simulink model "pointing_group24"  (R2023b)
settings: Solver=FixedStepAuto  StartTime=0.0  StopTime=T  RelTol=1e-3
values from neighbouring files (symbols this model uses):
  a = 6939    [Air_Drag_script.m]    (also in main.m = 6939.063; main_group24.m = 6978)
  AccMagn = 0.5    [main_group24.m]
  AccSunSens = 0.125    [main_group24.m]
  ARW = deg2rad(0.10)    [main_group24.m]
  by = 0.1    [main_group24.m]
  bz = 0.1    [main_group24.m]
  c = 2.99792*10^8    (= 299792000)    [main.m]    (also in main_group24.m = 299792458)
  Cd = 2.2    [main_group24.m]
  e = 0    [Air_Drag_script.m]    (also in main.m = 0.001304; main_group24.m)
  G = [gn, gm, gvali, gsvi]    [main.m]    (also in main_group24.m)
  GyroSampleRate = 10    [main_group24.m]
  H = [hn, hm, hvali, hsvi]    [main.m]    (also in main_group24.m)
  H_0 = ((g1_0^2)+(g1_1^2)+(h1_1^2))^0.5    (= 2.98059244128e-05)    [main_group24.m]
  i = deg2rad(97.5307)    [Air_Drag_script.m]    (also in main.m; main_group24.m = deg2rad(98))
  I_tot = [Ix 0 0; 0 Iy 0; 0 0 Iz]    [data_mass.m]    (also in main_group24.m)
  invI_tot = inv(I_tot)    [data_mass.m]    (also in main_group24.m)
  Ix = J(1,1)    [Air_Drag_script.m]    (also in data_mass.m = 0.0755003333333; main.m = 0.057749855; main_group24.m = 0.0755003333333)
  Iy = J(2,2)    [Air_Drag_script.m]    (also in data_mass.m = 0.0755003333333; main.m = 0.04143542; main_group24.m = 0.0755003333333)
  Iz = J(3,3)    [Air_Drag_script.m]    (also in data_mass.m = 0.055; main.m = 0.024624309; main_group24.m = 0.055)
  k1 = 5e-2    (= 0.05)    [main_group24.m]
  k2 = 2.5e-2    (= 0.025)    [main_group24.m]
  m = [0.1; 0.1; 0.1]    [main.m]    (also in main_group24.m)
  MB = [4; 0.1; 0.1; 0.3]    [main.m]    (also in main_group24.m)
  MMnoise = 15e-9*[1; 1; 1]    [main_group24.m]
  MMSampleRate = 1    [main_group24.m]
  mu = 3.98600433e+5    (= 398600.433)    [main.m]    (also in main_group24.m)
  n = 0.0011    [Air_Drag_script.m]    (also in main.m = sqrt(mu/a^3); main_group24.m = sqrt(mu/a^3))
  n_E = 729.2e-07    (= 7.292e-05)    [main_group24.m]
  om_E = 0.000072921    (= 7.2921e-05)    [main_group24.m]
  P = Fe/c    (= 4.52980041279e-06)    [main_group24.m]
  q0 = [ 1 1 1 1 ]'    [Air_Drag_script.m]    (also in main_group24.m = [0 0 0 1]')
  R_e = 6378    [main.m]    (also in main_group24.m)
  rho_air = 1.65e-13    [Air_Drag_script.m]    (also in main_group24.m = 6.967e-13)
  rho_d_body = 0.1*2/3    (= 0.0666666666667)    [main_group24.m]
  rho_d_sp = 0.1*2/3    (= 0.0666666666667)    [main_group24.m]
  rho_s_body = 0.5    [main_group24.m]
  rho_s_sp = 0.1    [main_group24.m]
  RRW = deg2rad(0.3)    [main_group24.m]
  SP = [1; 0.3; 0.1; 0.01]    [main.m]    (also in main_group24.m = [0.25; 0.1; 0.3; 0.01])
undefined symbols (not defined in the file or in its folder): pan, s1, s2, s3, s4, s5, s6, thrust
libraries: vrlib x25, matrix_library x17, simulink_extras x8, sharedutil x3, simulink x1
(part 3 of 5)

== system pointing_group24/Desturbances/External Torques/Reflected radiation/Force MB/Subsystem ==
  S_B : Inport
  N_MB : Inport  Port=2
  Constant3 : Constant  Value=[1, 1, 1]
  Matrix Multiply5 : Product  Multiplication=Matrix(*)
  Product10 : Product
  Reshape11 : Reshape  OutputDimensionality=Row vector (2-D)
  Reshape12 : Reshape  OutputDimensionality=Column vector (2-D)
  Sum of Elements : Sum  Inputs=+  CollapseMode=Specified dimension  CollapseDim=2
  Out1 : Outport
  wires:
  Reshape11/1 -> Matrix Multiply5/2
  Constant3/1 -> Reshape11/1
  Sum of Elements/1 -> Out1/1
  N_MB/1 -> Product10/2
  Product10/1 -> Sum of Elements/1
  S_B/1 -> Reshape12/1
  Reshape12/1 -> Matrix Multiply5/1
  Matrix Multiply5/1 -> Product10/1

== system pointing_group24/Desturbances/External Torques/Reflected radiation/SP center arm/r_SPx ==
  b_SP : Inport
  a_MB : Inport  Port=2
  Constant : Constant  Value=[1 0 0]
  Gain : Gain  Gain=1/2
  Gain1 : Gain  Gain=1/2
  Gain2 : Gain  Gain=-1
  Product : Product
  Reshape : Reshape  OutputDimensionality=Column vector (2-D)
  Sum : Sum
  r_SP1 : Outport
  r_SP2 : Outport  Port=2
  wires:
  Product/1 -> Gain2/1, r_SP1/1
  Gain2/1 -> r_SP2/1
  Sum/1 -> Product/2
  Reshape/1 -> Product/1
  Gain/1 -> Sum/2
  Gain1/1 -> Sum/1
  b_SP/1 -> Gain1/1
  a_MB/1 -> Gain/1
  Constant/1 -> Reshape/1

== system pointing_group24/Desturbances/External Torques/Reflected radiation/SP center arm/r_SPy ==
  b_SP : Inport
  b_MB : Inport  Port=2
  Constant : Constant  Value=[0 1 0]
  Gain : Gain  Gain=1/2
  Gain1 : Gain  Gain=1/2
  Gain2 : Gain  Gain=-1
  Product : Product
  Reshape : Reshape  OutputDimensionality=Column vector (2-D)
  Sum : Sum
  r_SP1 : Outport
  r_SP2 : Outport  Port=2
  wires:
  Constant/1 -> Reshape/1
  b_MB/1 -> Gain/1
  b_SP/1 -> Gain1/1
  Gain1/1 -> Sum/1
  Gain/1 -> Sum/2
  Reshape/1 -> Product/1
  Sum/1 -> Product/2
  Gain2/1 -> r_SP2/1
  Product/1 -> r_SP1/1, Gain2/1

== system pointing_group24/Desturbances/External Torques/Reflected radiation/S_B dot N_MB/If Action Subsystem ==
  NMB : Inport
  Action Port : ActionPort  ActionPortLabel=if(u1 > 0)
  Constant : Constant
  Selector : Selector  NumberOfDimensions=2  InputPortWidth=3  IndexOptions=Index vector (dialog),Index vector (dialog)  Indices=1,[1 2 3]  OutputSizes=1,1
  x : Outport
  pointer : Outport  Port=2
  wires:
  Constant/1 -> pointer/1
  Selector/1 -> x/1
  NMB/1 -> Selector/1

== system pointing_group24/Desturbances/External Torques/Reflected radiation/S_B dot N_MB/If Action Subsystem1 ==
  NMB : Inport
  Action Port : ActionPort  ActionPortLabel=if(u1 > 0)
  Constant : Constant
  Selector : Selector  NumberOfDimensions=2  InputPortWidth=3  IndexOptions=Index vector (dialog),Index vector (dialog)  Indices=2,[1 2 3]  OutputSizes=1,1
  y : Outport
  pointer : Outport  Port=2
  wires:
  Constant/1 -> pointer/1
  NMB/1 -> Selector/1
  Selector/1 -> y/1

== system pointing_group24/Desturbances/External Torques/Reflected radiation/S_B dot N_MB/If Action Subsystem2 ==
  NMB : Inport
  Action Port : ActionPort  ActionPortLabel=if(u1 > 0)
  Constant : Constant
  Selector : Selector  NumberOfDimensions=2  InputPortWidth=3  IndexOptions=Index vector (dialog),Index vector (dialog)  Indices=3,[1 2 3]  OutputSizes=1,1
  z : Outport
  pointer : Outport  Port=2
  wires:
  Constant/1 -> pointer/1
  Selector/1 -> z/1
  NMB/1 -> Selector/1

== system pointing_group24/Desturbances/External Torques/Reflected radiation/S_B dot N_MB/If Action Subsystem3 ==
  NMB : Inport
  Action Port : ActionPort  ActionPortLabel=else
  Constant : Constant  Value=-1
  Selector : Selector  NumberOfDimensions=2  InputPortWidth=3  IndexOptions=Index vector (dialog),Index vector (dialog)  Indices=4,[1 2 3]  OutputSizes=1,1
  -x : Outport
  pointer : Outport  Port=2
  wires:
  Constant/1 -> pointer/1
  NMB/1 -> Selector/1
  Selector/1 -> -x/1

== system pointing_group24/Desturbances/External Torques/Reflected radiation/S_B dot N_MB/If Action Subsystem4 ==
  NMB : Inport
  Action Port : ActionPort  ActionPortLabel=else
  Constant : Constant  Value=-1
  Selector : Selector  NumberOfDimensions=2  InputPortWidth=3  IndexOptions=Index vector (dialog),Index vector (dialog)  Indices=5,[1 2 3]  OutputSizes=1,1
  -y : Outport
  pointer : Outport  Port=2
  wires:
  Constant/1 -> pointer/1
  Selector/1 -> -y/1
  NMB/1 -> Selector/1

== system pointing_group24/Desturbances/External Torques/Reflected radiation/S_B dot N_MB/If Action Subsystem5 ==
  NMB : Inport
  Action Port : ActionPort  ActionPortLabel=else
  Constant : Constant  Value=-1
  Selector : Selector  NumberOfDimensions=2  InputPortWidth=3  IndexOptions=Index vector (dialog),Index vector (dialog)  Indices=6,[1 2 3]  OutputSizes=1,1
  -z : Outport
  pointer : Outport  Port=2
  wires:
  Constant/1 -> pointer/1
  NMB/1 -> Selector/1
  Selector/1 -> -z/1

== system pointing_group24/Desturbances/External Torques/Reflected radiation/S_B dot N_SP/If Action Subsystem ==
  N_SP : Inport
  Action Port : ActionPort  ActionPortLabel=if(u1 > 0)
  Constant : Constant
  Selector : Selector  NumberOfDimensions=2  InputPortWidth=3  IndexOptions=Index vector (dialog),Index vector (dialog)  Indices=1,[1 2 3]  OutputSizes=1,1
  true_NSP : Outport
  pointer : Outport  Port=2
  wires:
  Selector/1 -> true_NSP/1
  Constant/1 -> pointer/1
  N_SP/1 -> Selector/1

== system pointing_group24/Desturbances/External Torques/Reflected radiation/S_B dot N_SP/If Action Subsystem1 ==
  N_SP : Inport
  Action Port : ActionPort  ActionPortLabel=if(u1 > 0)
  Constant : Constant  Value=-1
  Selector : Selector  NumberOfDimensions=2  InputPortWidth=3  IndexOptions=Index vector (dialog),Index vector (dialog)  Indices=2,[1 2 3]  OutputSizes=1,1
  true_NSP : Outport
  pointer : Outport  Port=2
  wires:
  N_SP/1 -> Selector/1
  Constant/1 -> pointer/1
  Selector/1 -> true_NSP/1

== system pointing_group24/Desturbances/External Torques/Reflected radiation/Torque arm MB/creazione raggi vettore tra CM MB e centro facce illuminate della faccia che ha come normale l'asse i ==
  S_B : Inport
  MB : Inport  Port=2
  A_vect : Inport  Port=3
  pointer : Inport  Port=4
  Add2 : Sum  Inputs=+|+|+|+|+
  Demux1 : Demux  Outputs=3
  If Action Subsystem : Subsystem  TreatAsAtomicUnit=on
  If Action Subsystem1 : Subsystem  TreatAsAtomicUnit=on
  If Action Subsystem2 : Subsystem  TreatAsAtomicUnit=on
  If Action Subsystem3 : Subsystem  TreatAsAtomicUnit=on
  If Action Subsystem4 : Subsystem  TreatAsAtomicUnit=on
  If Action Subsystem5 : Subsystem  TreatAsAtomicUnit=on
  If Action Subsystem6 : Subsystem  TreatAsAtomicUnit=on
  If Action Subsystem8 : Subsystem  TreatAsAtomicUnit=on
  If1 : If  NumInputs=2  IfExpression=u1>0 & u2>0
  If2 : If  NumInputs=2  IfExpression=u1<0 & u2>0
  If3 : If  NumInputs=2  IfExpression=u1>0 & u2<0
  If4 : If  NumInputs=2  IfExpression=u1<0 & u2<0
  Merge{,1..3} (4 alike) : Merge
  Reshape1 : Reshape  OutputDimensionality=Column vector (2-D)
  Terminator1 : Terminator
  creating distance between cm MB and centro geom lato : Subsystem
  Out1 : Outport
  wires:
  pointer/1 -> creating distance between cm MB and centro geom lato/2(pointer)
  A_vect/1 -> [A_vect]
  [MB] -> creating distance between cm MB and centro geom lato/1(MB)
  If Action Subsystem6/1(Out1) -> Merge3/2
  Merge2/1 -> Add2/4  "raggio vettore centro geom lato- centro geom lato illuminato"
  If Action Subsystem5/1(Out1) -> Merge2/2
  If Action Subsystem1/1(r_cface_cluce_yneg_z_pos) -> Merge2/1
  If Action Subsystem3/1(Out1) -> Merge1/2
  If4/2 -> If Action Subsystem6/Action
  If3/2 -> If Action Subsystem5/Action
  If2/2 -> If Action Subsystem3/Action
  If Action Subsystem8/1(Out1) -> Merge/2
  [MB] -> If Action Subsystem2/2(MB)
  [MB] -> If Action Subsystem1/2(MB)
  [MB] -> If Action Subsystem4/2(MB)
  [MB] -> If Action Subsystem/2(MB)
  MB/1 -> [MB]
  Demux1/1 -> Terminator1/1  "S_B_x"
  creating distance between cm MB and centro geom lato/1(Out1) -> Add2/1
  Demux1/3 -> If1/1, If2/1, If3/1, If4/1  "S_B_z"
  If1/1 -> If Action Subsystem/Action
  If2/1 -> If Action Subsystem4/Action
  Demux1/2 -> If1/2, If4/2, If3/2, If2/2  "S_B_y"
  Reshape1/1 -> Demux1/1
  S_B/1 -> Reshape1/1
  If1/2 -> If Action Subsystem8/Action
  If Action Subsystem/1(r_cface_cluce_yz_pos) -> Merge/1
  Merge/1 -> Add2/2  "raggio vettore centro geom lato- centro geom lato illuminato"
  If Action Subsystem4/1(r_cface_cluce_zneg_y_pos) -> Merge1/1
  Merge1/1 -> Add2/3  "raggio vettore centro geom lato- centro geom lato illuminato"
  [A_vect] -> If Action Subsystem/1(Areas_vect)
  If3/1 -> If Action Subsystem1/Action
  If Action Subsystem2/1(r_cface_cluce_yneg_z_neg) -> Merge3/1
  If4/1 -> If Action Subsystem2/Action
  Merge3/1 -> Add2/5  "raggio vettore centro geom lato- centro geom lato illuminato"
  Add2/1 -> Out1/1
  [A_vect] -> If Action Subsystem4/1(Areas_vect)
  [A_vect] -> If Action Subsystem1/1(Areas_vect)
  [A_vect] -> If Action Subsystem2/1(Areas_vect)

== system pointing_group24/Desturbances/External Torques/Reflected radiation/Torque arm MB/creazione raggi vettore tra CM MB e centro facce illuminate della faccia che ha come normale l'asse j ==
  S_B : Inport
  MB : Inport  Port=2
  A_vect : Inport  Port=3
  pointer : Inport  Port=4
  Add2 : Sum  Inputs=+|+|+|+|+
  Demux1 : Demux  Outputs=3
  If Action Subsystem : Subsystem  TreatAsAtomicUnit=on
  If Action Subsystem1 : Subsystem  TreatAsAtomicUnit=on
  If Action Subsystem2 : Subsystem  TreatAsAtomicUnit=on
  If Action Subsystem3 : Subsystem  TreatAsAtomicUnit=on
  If Action Subsystem4 : Subsystem  TreatAsAtomicUnit=on
  If Action Subsystem5 : Subsystem  TreatAsAtomicUnit=on
  If Action Subsystem6 : Subsystem  TreatAsAtomicUnit=on
  If Action Subsystem7 : Subsystem  TreatAsAtomicUnit=on
  If1 : If  NumInputs=2  IfExpression=u1>0 & u2>0
  If2 : If  NumInputs=2  IfExpression=u1<0 & u2>0
  If3 : If  NumInputs=2  IfExpression=u1>0 & u2<0
  If4 : If  NumInputs=2  IfExpression=u1<0 & u2<0
  Merge{,1..3} (4 alike) : Merge
  Reshape1 : Reshape  OutputDimensionality=Column vector (2-D)
  Terminator1 : Terminator
  creating distance between cm MB and centro geom lato1 : Subsystem
  Out1 : Outport
  wires:
  pointer/1 -> creating distance between cm MB and centro geom lato1/2(pointer)
  A_vect/1 -> [A_vect]
  [MB] -> creating distance between cm MB and centro geom lato1/1(MB)
  If Action Subsystem7/1(Out1) -> Merge3/2
  If Action Subsystem6/1(Out1) -> Merge2/2
  If Action Subsystem2/1(r_cface_cluce_x_neg_z_pos) -> Merge2/1
  If Action Subsystem4/1(Out1) -> Merge1/2
  If Action Subsystem5/1(Out1) -> Merge/2
  If4/2 -> If Action Subsystem7/Action
  If3/2 -> If Action Subsystem6/Action
  If2/2 -> If Action Subsystem4/Action
  If1/2 -> If Action Subsystem5/Action
  [MB] -> If Action Subsystem3/2(MB)
  [MB] -> If Action Subsystem2/2(MB)
  [MB] -> If Action Subsystem1/2(MB)
  [MB] -> If Action Subsystem/2(MB)
  MB/1 -> [MB]
  Demux1/1 -> If2/2, If3/2, If4/2, If1/2  "S_B_x"
  Demux1/3 -> If1/1, If2/1, If3/1, If4/1  "S_B_z"
  [A_vect] -> If Action Subsystem3/1(Areas_vect)
  [A_vect] -> If Action Subsystem2/1(Areas_vect)
  [A_vect] -> If Action Subsystem1/1(Areas_vect)
  Add2/1 -> Out1/1
  Merge3/1 -> Add2/5  "raggio vettore centro geom lato- centro geom lato illuminato"
  If4/1 -> If Action Subsystem3/Action
  If Action Subsystem3/1(r_cface_cluce_x_neg_z_neg) -> Merge3/1
  If3/1 -> If Action Subsystem2/Action
  Merge2/1 -> Add2/4  "raggio vettore centro geom lato- centro geom lato illuminato"
  [A_vect] -> If Action Subsystem/1(Areas_vect)
  Merge1/1 -> Add2/3  "raggio vettore centro geom lato- centro geom lato illuminato"
  If Action Subsystem1/1(r_cface_cluce_x_pos_z_neg) -> Merge1/1
  Merge/1 -> Add2/2  "raggio vettore centro geom lato- centro geom lato illuminato"
  If Action Subsystem/1(r_cface_cluce_xz_pos) -> Merge/1
  S_B/1 -> Reshape1/1
  Reshape1/1 -> Demux1/1
  If2/1 -> If Action Subsystem1/Action
  If1/1 -> If Action Subsystem/Action
  creating distance between cm MB and centro geom lato1/1(Out1) -> Add2/1
  Demux1/2 -> Terminator1/1

== system pointing_group24/Desturbances/External Torques/Reflected radiation/Torque arm MB/creazione raggi vettore tra CM MB e centro facce illuminate della faccia che ha come normale l'asse k ==
  S_B : Inport
  MB : Inport  Port=2
  A_vect : Inport  Port=3
  pointer : Inport  Port=4
  Add2 : Sum  Inputs=+|+|+|+|+
  Demux1 : Demux  Outputs=3
  If Action Subsystem : Subsystem  TreatAsAtomicUnit=on
  If Action Subsystem1 : Subsystem  TreatAsAtomicUnit=on
  If Action Subsystem2 : Subsystem  TreatAsAtomicUnit=on
  If Action Subsystem3 : Subsystem  TreatAsAtomicUnit=on
  If Action Subsystem4 : Subsystem  TreatAsAtomicUnit=on
  If Action Subsystem5 : Subsystem  TreatAsAtomicUnit=on
  If Action Subsystem6 : Subsystem  TreatAsAtomicUnit=on
  If Action Subsystem7 : Subsystem  TreatAsAtomicUnit=on
  If1 : If  NumInputs=2  IfExpression=u1>0 & u2>0
  If2 : If  NumInputs=2  IfExpression=u1<0 & u2>0
  If3 : If  NumInputs=2  IfExpression=u1>0 & u2<0
  If4 : If  NumInputs=2  IfExpression=u1<0 & u2<0
  Merge{,1..3} (4 alike) : Merge
  Reshape1 : Reshape  OutputDimensionality=Column vector (2-D)
  Terminator1 : Terminator
  creating distance between cm MB and centro geom lato1 : Subsystem
  Out1 : Outport
  wires:
  pointer/1 -> creating distance between cm MB and centro geom lato1/2(pointer)
  A_vect/1 -> [A_vect]
  creating distance between cm MB and centro geom lato1/1(Out1) -> Add2/1
  [MB] -> creating distance between cm MB and centro geom lato1/1(MB)
  If Action Subsystem7/1(Out1) -> Merge3/2
  If Action Subsystem2/1(r_cface_cluce_xneg_y_neg) -> Merge3/1
  If Action Subsystem6/1(Out1) -> Merge2/2
  If Action Subsystem3/1(Out1) -> Merge1/2
  If Action Subsystem4/1(r_cface_cluce_xneg_y_pos) -> Merge1/1
  If Action Subsystem5/1(Out1) -> Merge/2
  If Action Subsystem/1(r_cface_cluce_xy_pos) -> Merge/1
  If2/2 -> If Action Subsystem3/Action
  [MB] -> If Action Subsystem2/2(MB1)
  [MB] -> If Action Subsystem1/2(MB)
  [MB] -> If Action Subsystem4/2(MB1)
  [MB] -> If Action Subsystem/2(MB)
  MB/1 -> [MB]
  [A_vect] -> If Action Subsystem2/1(Areas_vect)
  [A_vect] -> If Action Subsystem1/1(Areas_vect)
  [A_vect] -> If Action Subsystem4/1(Areas_vect)
  Add2/1 -> Out1/1
  Merge3/1 -> Add2/5  "raggio vettore centro geom lato- centro geom lato illuminato"
  If4/1 -> If Action Subsystem2/Action
  If4/2 -> If Action Subsystem7/Action
  If3/1 -> If Action Subsystem1/Action
  If Action Subsystem1/1(r_cface_cluce_xpos_y_neg) -> Merge2/1
  If3/2 -> If Action Subsystem6/Action
  Merge2/1 -> Add2/4  "raggio vettore centro geom lato- centro geom lato illuminato"
  [A_vect] -> If Action Subsystem/1(Areas_vect)
  Merge1/1 -> Add2/3  "raggio vettore centro geom lato- centro geom lato illuminato"
  Merge/1 -> Add2/2  "raggio vettore centro geom lato- centro geom lato illuminato"
  If1/2 -> If Action Subsystem5/Action
  S_B/1 -> Reshape1/1
  Reshape1/1 -> Demux1/1
  Demux1/2 -> If1/2, If2/2, If3/2, If4/2  "S_B_y"
  If2/1 -> If Action Subsystem4/Action
  If1/1 -> If Action Subsystem/Action
  Demux1/1 -> If2/1, If3/1, If4/1, If1/1  "S_B_x"
  Demux1/3 -> Terminator1/1

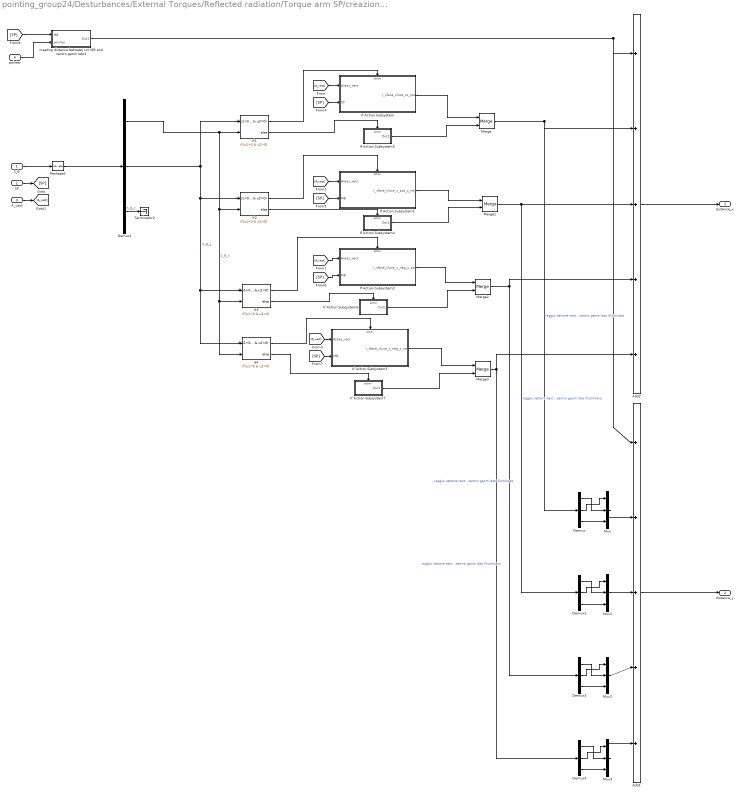
== system pointing_group24/Desturbances/External Torques/Reflected radiation/Torque arm SP/creazione raggi vettore tra CM SP e centro di pressione della faccia illuminata ==
  S_B : Inport
  SP : Inport  Port=2
  A_vect : Inport  Port=3
  pointer : Inport  Port=4
  Add1 : Sum  Inputs=+|+|+|+|+
  Add2 : Sum  Inputs=+|+|+|+|+
  Demux{,1..4} (5 alike) : Demux  Outputs=3
  If Action Subsystem : Subsystem  TreatAsAtomicUnit=on
  If Action Subsystem1 : Subsystem  TreatAsAtomicUnit=on
  If Action Subsystem2 : Subsystem  TreatAsAtomicUnit=on
  If Action Subsystem3 : Subsystem  TreatAsAtomicUnit=on
  If Action Subsystem4 : Subsystem  TreatAsAtomicUnit=on
  If Action Subsystem5 : Subsystem  TreatAsAtomicUnit=on
  If Action Subsystem6 : Subsystem  TreatAsAtomicUnit=on
  If Action Subsystem7 : Subsystem  TreatAsAtomicUnit=on
  If1 : If  NumInputs=2  IfExpression=u1>0 & u2>0
  If2 : If  NumInputs=2  IfExpression=u1<0 & u2>0
  If3 : If  NumInputs=2  IfExpression=u1>0 & u2<0
  If4 : If  NumInputs=2  IfExpression=u1<0 & u2<0
  Merge{,1..3} (4 alike) : Merge
  Mux{,1..3} (4 alike) : Mux  Inputs=3
  Reshape1 : Reshape  OutputDimensionality=Column vector (2-D)
  Terminator2 : Terminator
  creating distance between cm MB and centro geom lato1 : Subsystem
  distance_x : Outport
  distance_y : Outport  Port=2
  wires:
  Mux2/1 -> Add1/4
  Mux3/1 -> Add1/5
  Demux4/1 -> Mux3/2
  Demux4/2 -> Mux3/1
  Demux4/3 -> Mux3/3
  Demux3/3 -> Mux2/3
  Demux3/2 -> Mux2/1
  Demux3/1 -> Mux2/2
  Demux2/1 -> Mux1/2
  Demux2/2 -> Mux1/1
  Demux2/3 -> Mux1/3
  Mux1/1 -> Add1/3
  Mux/1 -> Add1/2
  Demux/3 -> Mux/3
  Demux/2 -> Mux/1
  Demux/1 -> Mux/2
  Add1/1 -> distance_y/1
  Demux1/3 -> Terminator2/1  "S_B_z"
  pointer/1 -> creating distance between cm MB and centro geom lato1/2(pointer)
  A_vect/1 -> [A_vect]
  [SP] -> creating distance between cm MB and centro geom lato1/1(MB)
  If Action Subsystem7/1(Out1) -> Merge3/2
  If Action Subsystem6/1(Out1) -> Merge2/2
  If Action Subsystem2/1(r_cface_cluce_x_neg_z_pos) -> Merge2/1
  If Action Subsystem4/1(Out1) -> Merge1/2
  If Action Subsystem5/1(Out1) -> Merge/2
  If4/2 -> If Action Subsystem7/Action
  If3/2 -> If Action Subsystem6/Action
  If2/2 -> If Action Subsystem4/Action
  If1/2 -> If Action Subsystem5/Action
  [SP] -> If Action Subsystem3/2(MB)
  [SP] -> If Action Subsystem2/2(MB)
  [SP] -> If Action Subsystem1/2(MB)
  [SP] -> If Action Subsystem/2(SP)
  SP/1 -> [SP]
  Demux1/1 -> If2/2, If3/2, If4/2, If1/2  "S_B_x"
  Demux1/2 -> If1/1, If2/1, If3/1, If4/1  "S_B_y"
  [A_vect] -> If Action Subsystem3/1(Areas_vect)
  [A_vect] -> If Action Subsystem2/1(Areas_vect)
  [A_vect] -> If Action Subsystem1/1(Areas_vect)
  Add2/1 -> distance_x/1
  Merge3/1 -> Add2/5, Demux4/1  "raggio vettore centro geom lato- centro geom lato illuminato"
  If4/1 -> If Action Subsystem3/Action
  If Action Subsystem3/1(r_cface_cluce_x_neg_z_neg) -> Merge3/1
  If3/1 -> If Action Subsystem2/Action
  Merge2/1 -> Add2/4, Demux3/1  "raggio vettore centro geom lato- centro geom lato illuminato"
  [A_vect] -> If Action Subsystem/1(Areas_vect)
  Merge1/1 -> Add2/3, Demux2/1  "raggio vettore centro geom lato- centro geom lato illuminato"
  If Action Subsystem1/1(r_cface_cluce_x_pos_z_neg) -> Merge1/1
  Merge/1 -> Add2/2, Demux/1  "raggio vettore centro geom lato- centro geom lato illuminato"
  If Action Subsystem/1(r_cface_cluce_xz_pos) -> Merge/1
  S_B/1 -> Reshape1/1
  Reshape1/1 -> Demux1/1
  If2/1 -> If Action Subsystem1/Action
  If1/1 -> If Action Subsystem/Action
  creating distance between cm MB and centro geom lato1/1(Out1) -> Add2/1, Add1/1

== system pointing_group24/Desturbances/External Torques/SRP con frecce/SRP/Subsystem ==
  S_B : Inport
  Add22 : Sum
  Add23 : Sum
  Add24 : Sum  Inputs=+-
  Constant30 : Constant  Value=s2.A
  Constant31 : Constant  Value=s2.n
  Constant44 : Constant  Value=rho_d_body
  Constant47 : Constant  Value=s2.n
  Constant50 : Constant
  Constant51 : Constant  Value=rho_s_body
  Constant52 : Constant  Value=s2.r
  Cross Product10 : vrlib/Utilities/Cross Product
  Dot Product10 : DotProduct  OutDataTypeStr=Inherit: Inherit via internal rule
  Gain40 : Gain  Gain=0
  Gain41 : Gain  Gain=-P
  Gain42 : Gain  Gain=2
  Gain43 : Gain  Gain=rho_s_body
  Product{1..4} (4 alike) : Product
  Switch10 : Switch  Criteria=u2 > Threshold  SaturateOnIntegerOverflow=off  InputSameDT=off
  pan2 : Outport
  wires:
  Constant50/1 -> Add24/1
  Gain42/1 -> Gain43/1
  Cross Product10/1 -> pan2/1
  Gain43/1 -> Add22/2
  Constant52/1 -> Cross Product10/1
  Add22/1 -> Product2/2
  Gain41/1 -> Product1/2
  Gain40/1 -> Switch10/3
  Dot Product10/1 -> Gain40/1, Switch10/1, Switch10/2
  Product2/1 -> Add23/2
  Constant31/1 -> Dot Product10/2
  Constant51/1 -> Add24/2
  Add24/1 -> Product3/2
  Product3/1 -> Add23/1
  Constant44/1 -> Add22/1
  S_B/1 -> Product3/1, Dot Product10/1
  Product1/1 -> Product4/1
  Constant47/1 -> Product2/1
  Switch10/1 -> Gain41/1, Gain42/1
  Constant30/1 -> Product1/1
  Product4/1 -> Cross Product10/2
  Add23/1 -> Product4/2

== system pointing_group24/Desturbances/External Torques/SRP con frecce/SRP/Subsystem1 ==
  S_B : Inport
  Add22 : Sum
  Add23 : Sum
  Add24 : Sum  Inputs=+-
  Constant30 : Constant  Value=s3.A
  Constant31 : Constant  Value=s3.n
  Constant44 : Constant  Value=rho_d_body
  Constant47 : Constant  Value=s3.n
  Constant50 : Constant
  Constant51 : Constant  Value=rho_s_body
  Constant52 : Constant  Value=s3.r
  Cross Product10 : vrlib/Utilities/Cross Product
  Dot Product10 : DotProduct  OutDataTypeStr=Inherit: Inherit via internal rule
  Gain40 : Gain  Gain=0
  Gain41 : Gain  Gain=-P
  Gain42 : Gain  Gain=2
  Gain43 : Gain  Gain=rho_s_body
  Product{1..4} (4 alike) : Product
  Switch10 : Switch  Criteria=u2 > Threshold  SaturateOnIntegerOverflow=off  InputSameDT=off
  pan3 : Outport
  wires:
  Add23/1 -> Product4/2
  Product4/1 -> Cross Product10/2
  Constant30/1 -> Product1/1
  Switch10/1 -> Gain42/1, Gain41/1
  Constant47/1 -> Product2/1
  Product1/1 -> Product4/1
  S_B/1 -> Dot Product10/1, Product3/1
  Constant44/1 -> Add22/1
  Product3/1 -> Add23/1
  Add24/1 -> Product3/2
  Constant51/1 -> Add24/2
  Constant31/1 -> Dot Product10/2
  Product2/1 -> Add23/2
  Dot Product10/1 -> Switch10/2, Switch10/1, Gain40/1
  Gain40/1 -> Switch10/3
  Gain41/1 -> Product1/2
  Add22/1 -> Product2/2
  Constant52/1 -> Cross Product10/1
  Gain43/1 -> Add22/2
  Cross Product10/1 -> pan3/1
  Gain42/1 -> Gain43/1
  Constant50/1 -> Add24/1

== system pointing_group24/Desturbances/External Torques/SRP con frecce/SRP/Subsystem2 ==
  S_B : Inport
  Add22 : Sum
  Add23 : Sum
  Add24 : Sum  Inputs=+-
  Constant30 : Constant  Value=s1.A
  Constant31 : Constant  Value=s1.n
  Constant44 : Constant  Value=rho_d_body
  Constant47 : Constant  Value=s1.n
  Constant50 : Constant
  Constant51 : Constant  Value=rho_s_body
  Constant52 : Constant  Value=s1.r
  Cross Product10 : vrlib/Utilities/Cross Product
  Dot Product10 : DotProduct  OutDataTypeStr=Inherit: Inherit via internal rule
  Gain40 : Gain  Gain=0
  Gain41 : Gain  Gain=-P
  Gain42 : Gain  Gain=2
  Gain43 : Gain  Gain=rho_s_body
  Product{1..4} (4 alike) : Product
  Switch10 : Switch  Criteria=u2 > Threshold  SaturateOnIntegerOverflow=off  InputSameDT=off
  pan1 : Outport
  wires:
  Add23/1 -> Product4/2
  Product4/1 -> Cross Product10/2
  Constant30/1 -> Product1/1
  Switch10/1 -> Gain42/1, Gain41/1
  Constant47/1 -> Product2/1
  Product1/1 -> Product4/1
  S_B/1 -> Dot Product10/1, Product3/1
  Constant44/1 -> Add22/1
  Product3/1 -> Add23/1
  Add24/1 -> Product3/2
  Constant51/1 -> Add24/2
  Constant31/1 -> Dot Product10/2
  Product2/1 -> Add23/2
  Dot Product10/1 -> Switch10/2, Switch10/1, Gain40/1
  Gain40/1 -> Switch10/3
  Gain41/1 -> Product1/2
  Add22/1 -> Product2/2
  Constant52/1 -> Cross Product10/1
  Gain43/1 -> Add22/2
  Cross Product10/1 -> pan1/1
  Gain42/1 -> Gain43/1
  Constant50/1 -> Add24/1

== system pointing_group24/Desturbances/External Torques/SRP con frecce/SRP/Subsystem3 ==
  S_B : Inport
  Add22 : Sum
  Add23 : Sum
  Add24 : Sum  Inputs=+-
  Constant30 : Constant  Value=s5.A
  Constant31 : Constant  Value=s5.n
  Constant44 : Constant  Value=rho_d_body
  Constant47 : Constant  Value=s5.n
  Constant50 : Constant
  Constant51 : Constant  Value=rho_s_body
  Constant52 : Constant  Value=s5.r
  Cross Product10 : vrlib/Utilities/Cross Product
  Dot Product10 : DotProduct  OutDataTypeStr=Inherit: Inherit via internal rule
  Gain40 : Gain  Gain=0
  Gain41 : Gain  Gain=-P
  Gain42 : Gain  Gain=2
  Gain43 : Gain  Gain=rho_s_body
  Product{1..4} (4 alike) : Product
  Switch10 : Switch  Criteria=u2 > Threshold  SaturateOnIntegerOverflow=off  InputSameDT=off
  pan5 : Outport
  wires:
  Constant50/1 -> Add24/1
  Gain42/1 -> Gain43/1
  Cross Product10/1 -> pan5/1
  Gain43/1 -> Add22/2
  Constant52/1 -> Cross Product10/1
  Add22/1 -> Product2/2
  Gain41/1 -> Product1/2
  Gain40/1 -> Switch10/3
  Dot Product10/1 -> Gain40/1, Switch10/1, Switch10/2
  Product2/1 -> Add23/2
  Constant31/1 -> Dot Product10/2
  Constant51/1 -> Add24/2
  Add24/1 -> Product3/2
  Product3/1 -> Add23/1
  Constant44/1 -> Add22/1
  S_B/1 -> Product3/1, Dot Product10/1
  Product1/1 -> Product4/1
  Constant47/1 -> Product2/1
  Switch10/1 -> Gain41/1, Gain42/1
  Constant30/1 -> Product1/1
  Product4/1 -> Cross Product10/2
  Add23/1 -> Product4/2

== system pointing_group24/Desturbances/External Torques/SRP con frecce/SRP/Subsystem4 ==
  S_B : Inport
  Add22 : Sum
  Add23 : Sum
  Add24 : Sum  Inputs=+-
  Constant30 : Constant  Value=s4.A
  Constant31 : Constant  Value=s4.n
  Constant44 : Constant  Value=rho_d_body
  Constant47 : Constant  Value=s4.n
  Constant50 : Constant
  Constant51 : Constant  Value=rho_s_body
  Constant52 : Constant  Value=s4.r
  Cross Product10 : vrlib/Utilities/Cross Product
  Dot Product10 : DotProduct  OutDataTypeStr=Inherit: Inherit via internal rule
  Gain40 : Gain  Gain=0
  Gain41 : Gain  Gain=-P
  Gain42 : Gain  Gain=2
  Gain43 : Gain  Gain=rho_s_body
  Product{1..4} (4 alike) : Product
  Switch10 : Switch  Criteria=u2 > Threshold  SaturateOnIntegerOverflow=off  InputSameDT=off
  pan4 : Outport
  wires:
  Constant50/1 -> Add24/1
  Gain42/1 -> Gain43/1
  Cross Product10/1 -> pan4/1
  Gain43/1 -> Add22/2
  Constant52/1 -> Cross Product10/1
  Add22/1 -> Product2/2
  Gain41/1 -> Product1/2
  Gain40/1 -> Switch10/3
  Dot Product10/1 -> Gain40/1, Switch10/1, Switch10/2
  Product2/1 -> Add23/2
  Constant31/1 -> Dot Product10/2
  Constant51/1 -> Add24/2
  Add24/1 -> Product3/2
  Product3/1 -> Add23/1
  Constant44/1 -> Add22/1
  S_B/1 -> Product3/1, Dot Product10/1
  Product1/1 -> Product4/1
  Constant47/1 -> Product2/1
  Switch10/1 -> Gain41/1, Gain42/1
  Constant30/1 -> Product1/1
  Product4/1 -> Cross Product10/2
  Add23/1 -> Product4/2

== system pointing_group24/Desturbances/External Torques/SRP con frecce/SRP/Subsystem5 ==
  S_B : Inport
  Add22 : Sum
  Add23 : Sum
  Add24 : Sum  Inputs=+-
  Constant30 : Constant  Value=pan.A
  Constant31 : Constant  Value=pan.n1
  Constant44 : Constant  Value=rho_d_sp
  Constant47 : Constant  Value=pan.n1
  Constant50 : Constant
  Constant51 : Constant  Value=rho_s_sp
  Constant52 : Constant  Value=pan.r
  Cross Product10 : vrlib/Utilities/Cross Product
  Dot Product10 : DotProduct  OutDataTypeStr=Inherit: Inherit via internal rule
  Gain40 : Gain  Gain=0
  Gain41 : Gain  Gain=-P
  Gain42 : Gain  Gain=2
  Gain43 : Gain  Gain=rho_s_sp
  Product{1..4} (4 alike) : Product
  Switch10 : Switch  Criteria=u2 > Threshold  SaturateOnIntegerOverflow=off  InputSameDT=off
  ps1 : Outport
  wires:
  Add23/1 -> Product4/2
  Product4/1 -> Cross Product10/2
  Constant30/1 -> Product1/1
  Switch10/1 -> Gain42/1, Gain41/1
  Constant47/1 -> Product2/1
  Product1/1 -> Product4/1
  S_B/1 -> Dot Product10/1, Product3/1
  Constant44/1 -> Add22/1
  Product3/1 -> Add23/1
  Add24/1 -> Product3/2
  Constant51/1 -> Add24/2
  Constant31/1 -> Dot Product10/2
  Product2/1 -> Add23/2
  Dot Product10/1 -> Switch10/2, Switch10/1, Gain40/1
  Gain40/1 -> Switch10/3
  Gain41/1 -> Product1/2
  Add22/1 -> Product2/2
  Constant52/1 -> Cross Product10/1
  Gain43/1 -> Add22/2
  Cross Product10/1 -> ps1/1
  Gain42/1 -> Gain43/1
  Constant50/1 -> Add24/1

== system pointing_group24/Desturbances/External Torques/SRP con frecce/SRP/Subsystem6 ==
  S_B : Inport
  Add22 : Sum
  Add23 : Sum
  Add24 : Sum  Inputs=+-
  Constant30 : Constant  Value=pan.A
  Constant31 : Constant  Value=pan.n2
  Constant44 : Constant  Value=rho_d_sp
  Constant47 : Constant  Value=pan.n2
  Constant50 : Constant
  Constant51 : Constant  Value=rho_s_sp
  Constant52 : Constant  Value=pan.r
  Cross Product10 : vrlib/Utilities/Cross Product
  Dot Product10 : DotProduct  OutDataTypeStr=Inherit: Inherit via internal rule
  Gain40 : Gain  Gain=0
  Gain41 : Gain  Gain=-P
  Gain42 : Gain  Gain=2
  Gain43 : Gain  Gain=rho_s_sp
  Product{1..4} (4 alike) : Product
  Switch10 : Switch  Criteria=u2 > Threshold  SaturateOnIntegerOverflow=off  InputSameDT=off
  ps2 : Outport
  wires:
  Constant50/1 -> Add24/1
  Gain42/1 -> Gain43/1
  Cross Product10/1 -> ps2/1
  Gain43/1 -> Add22/2
  Constant52/1 -> Cross Product10/1
  Add22/1 -> Product2/2
  Gain41/1 -> Product1/2
  Gain40/1 -> Switch10/3
  Dot Product10/1 -> Gain40/1, Switch10/1, Switch10/2
  Product2/1 -> Add23/2
  Constant31/1 -> Dot Product10/2
  Constant51/1 -> Add24/2
  Add24/1 -> Product3/2
  Product3/1 -> Add23/1
  Constant44/1 -> Add22/1
  S_B/1 -> Product3/1, Dot Product10/1
  Product1/1 -> Product4/1
  Constant47/1 -> Product2/1
  Switch10/1 -> Gain41/1, Gain42/1
  Constant30/1 -> Product1/1
  Product4/1 -> Cross Product10/2
  Add23/1 -> Product4/2

== system pointing_group24/Desturbances/External Torques/SRP con frecce/SRP/Subsystem7 ==
  S_B : Inport
  Add22 : Sum
  Add23 : Sum
  Add24 : Sum  Inputs=+-
  Constant30 : Constant  Value=s6.A
  Constant31 : Constant  Value=s6.n
  Constant44 : Constant  Value=rho_d_body
  Constant47 : Constant  Value=s6.n
  Constant50 : Constant
  Constant51 : Constant  Value=rho_s_body
  Constant52 : Constant  Value=s6.r
  Cross Product10 : vrlib/Utilities/Cross Product
  Dot Product10 : DotProduct  OutDataTypeStr=Inherit: Inherit via internal rule
  Gain40 : Gain  Gain=0
  Gain41 : Gain  Gain=-P
  Gain42 : Gain  Gain=2
  Gain43 : Gain  Gain=rho_s_body
  Product{1..4} (4 alike) : Product
  Switch10 : Switch  Criteria=u2 > Threshold  SaturateOnIntegerOverflow=off  InputSameDT=off
  pan6 : Outport
  wires:
  Constant50/1 -> Add24/1
  Gain42/1 -> Gain43/1
  Cross Product10/1 -> pan6/1
  Gain43/1 -> Add22/2
  Constant52/1 -> Cross Product10/1
  Add22/1 -> Product2/2
  Gain41/1 -> Product1/2
  Gain40/1 -> Switch10/3
  Dot Product10/1 -> Gain40/1, Switch10/1, Switch10/2
  Product2/1 -> Add23/2
  Constant31/1 -> Dot Product10/2
  Constant51/1 -> Add24/2
  Add24/1 -> Product3/2
  Product3/1 -> Add23/1
  Constant44/1 -> Add22/1
  S_B/1 -> Product3/1, Dot Product10/1
  Product1/1 -> Product4/1
  Constant47/1 -> Product2/1
  Switch10/1 -> Gain41/1, Gain42/1
  Constant30/1 -> Product1/1
  Product4/1 -> Cross Product10/2
  Add23/1 -> Product4/2

== system pointing_group24/Desturbances/External Torques/Solar radiation/Force MB/Subsystem ==
  S_B : Inport
  N_MB : Inport  Port=2
  Constant3 : Constant  Value=[1, 1, 1]
  Matrix Multiply5 : Product  Multiplication=Matrix(*)
  Product10 : Product
  Reshape11 : Reshape  OutputDimensionality=Row vector (2-D)
  Reshape12 : Reshape  OutputDimensionality=Column vector (2-D)
  Sum of Elements : Sum  Inputs=+  CollapseMode=Specified dimension  CollapseDim=2
  Out1 : Outport
  wires:
  Matrix Multiply5/1 -> Product10/1
  Reshape12/1 -> Matrix Multiply5/1
  S_B/1 -> Reshape12/1
  Product10/1 -> Sum of Elements/1
  N_MB/1 -> Product10/2
  Sum of Elements/1 -> Out1/1
  Constant3/1 -> Reshape11/1
  Reshape11/1 -> Matrix Multiply5/2

== system pointing_group24/Desturbances/External Torques/Solar radiation/SP center arm/r_SPx ==
  b_SP : Inport
  a_MB : Inport  Port=2
  Constant : Constant  Value=[1 0 0]
  Gain : Gain  Gain=1/2
  Gain1 : Gain  Gain=1/2
  Gain2 : Gain  Gain=-1
  Product : Product
  Reshape : Reshape  OutputDimensionality=Column vector (2-D)
  Sum : Sum
  r_SP1 : Outport
  r_SP2 : Outport  Port=2
  wires:
  Constant/1 -> Reshape/1
  a_MB/1 -> Gain/1
  b_SP/1 -> Gain1/1
  Gain1/1 -> Sum/1
  Gain/1 -> Sum/2
  Reshape/1 -> Product/1
  Sum/1 -> Product/2
  Gain2/1 -> r_SP2/1
  Product/1 -> r_SP1/1, Gain2/1

== system pointing_group24/Desturbances/External Torques/Solar radiation/SP center arm/r_SPy ==
  b_SP : Inport
  b_MB : Inport  Port=2
  Constant : Constant  Value=[0 1 0]
  Gain : Gain  Gain=1/2
  Gain1 : Gain  Gain=1/2
  Gain2 : Gain  Gain=-1
  Product : Product
  Reshape : Reshape  OutputDimensionality=Column vector (2-D)
  Sum : Sum
  r_SP1 : Outport
  r_SP2 : Outport  Port=2
  wires:
  Product/1 -> Gain2/1, r_SP1/1
  Gain2/1 -> r_SP2/1
  Sum/1 -> Product/2
  Reshape/1 -> Product/1
  Gain/1 -> Sum/2
  Gain1/1 -> Sum/1
  b_SP/1 -> Gain1/1
  b_MB/1 -> Gain/1
  Constant/1 -> Reshape/1

== system pointing_group24/Desturbances/External Torques/Solar radiation/S_B dot N_MB/If Action Subsystem ==
  NMB : Inport
  Action Port : ActionPort  ActionPortLabel=if(u1 > 0)
  Constant : Constant
  Selector : Selector  NumberOfDimensions=2  InputPortWidth=3  IndexOptions=Index vector (dialog),Index vector (dialog)  Indices=1,[1 2 3]  OutputSizes=1,1
  x : Outport
  pointer : Outport  Port=2
  wires:
  NMB/1 -> Selector/1
  Selector/1 -> x/1
  Constant/1 -> pointer/1

== system pointing_group24/Desturbances/External Torques/Solar radiation/S_B dot N_MB/If Action Subsystem1 ==
  NMB : Inport
  Action Port : ActionPort  ActionPortLabel=if(u1 > 0)
  Constant : Constant
  Selector : Selector  NumberOfDimensions=2  InputPortWidth=3  IndexOptions=Index vector (dialog),Index vector (dialog)  Indices=2,[1 2 3]  OutputSizes=1,1
  y : Outport
  pointer : Outport  Port=2
  wires:
  Selector/1 -> y/1
  NMB/1 -> Selector/1
  Constant/1 -> pointer/1

== system pointing_group24/Desturbances/External Torques/Solar radiation/S_B dot N_MB/If Action Subsystem2 ==
  NMB : Inport
  Action Port : ActionPort  ActionPortLabel=if(u1 > 0)
  Constant : Constant
  Selector : Selector  NumberOfDimensions=2  InputPortWidth=3  IndexOptions=Index vector (dialog),Index vector (dialog)  Indices=3,[1 2 3]  OutputSizes=1,1
  z : Outport
  pointer : Outport  Port=2
  wires:
  NMB/1 -> Selector/1
  Selector/1 -> z/1
  Constant/1 -> pointer/1

== system pointing_group24/Desturbances/External Torques/Solar radiation/S_B dot N_MB/If Action Subsystem3 ==
  NMB : Inport
  Action Port : ActionPort  ActionPortLabel=else
  Constant : Constant  Value=-1
  Selector : Selector  NumberOfDimensions=2  InputPortWidth=3  IndexOptions=Index vector (dialog),Index vector (dialog)  Indices=4,[1 2 3]  OutputSizes=1,1
  -x : Outport
  pointer : Outport  Port=2
  wires:
  Selector/1 -> -x/1
  NMB/1 -> Selector/1
  Constant/1 -> pointer/1

== system pointing_group24/Desturbances/External Torques/Solar radiation/S_B dot N_MB/If Action Subsystem4 ==
  NMB : Inport
  Action Port : ActionPort  ActionPortLabel=else
  Constant : Constant  Value=-1
  Selector : Selector  NumberOfDimensions=2  InputPortWidth=3  IndexOptions=Index vector (dialog),Index vector (dialog)  Indices=5,[1 2 3]  OutputSizes=1,1
  -y : Outport
  pointer : Outport  Port=2
  wires:
  NMB/1 -> Selector/1
  Selector/1 -> -y/1
  Constant/1 -> pointer/1

== system pointing_group24/Desturbances/External Torques/Solar radiation/S_B dot N_MB/If Action Subsystem5 ==
  NMB : Inport
  Action Port : ActionPort  ActionPortLabel=else
  Constant : Constant  Value=-1
  Selector : Selector  NumberOfDimensions=2  InputPortWidth=3  IndexOptions=Index vector (dialog),Index vector (dialog)  Indices=6,[1 2 3]  OutputSizes=1,1
  -z : Outport
  pointer : Outport  Port=2
  wires:
  Selector/1 -> -z/1
  NMB/1 -> Selector/1
  Constant/1 -> pointer/1

== system pointing_group24/Desturbances/External Torques/Solar radiation/S_B dot N_SP/If Action Subsystem ==
  N_SP : Inport
  Action Port : ActionPort  ActionPortLabel=if(u1 > 0)
  Constant : Constant
  Selector : Selector  NumberOfDimensions=2  InputPortWidth=3  IndexOptions=Index vector (dialog),Index vector (dialog)  Indices=1,[1 2 3]  OutputSizes=1,1
  true_NSP : Outport
  pointer : Outport  Port=2
  wires:
  N_SP/1 -> Selector/1
  Constant/1 -> pointer/1
  Selector/1 -> true_NSP/1

== system pointing_group24/Desturbances/External Torques/Solar radiation/S_B dot N_SP/If Action Subsystem1 ==
  N_SP : Inport
  Action Port : ActionPort  ActionPortLabel=if(u1 > 0)
  Constant : Constant  Value=-1
  Selector : Selector  NumberOfDimensions=2  InputPortWidth=3  IndexOptions=Index vector (dialog),Index vector (dialog)  Indices=2,[1 2 3]  OutputSizes=1,1
  true_NSP : Outport
  pointer : Outport  Port=2
  wires:
  Selector/1 -> true_NSP/1
  Constant/1 -> pointer/1
  N_SP/1 -> Selector/1

== system pointing_group24/Desturbances/External Torques/Solar radiation/Torque arm MB/creazione raggi vettore tra CM MB e centro facce illuminate della faccia che ha come normale l'asse i ==
  S_B : Inport
  MB : Inport  Port=2
  A_vect : Inport  Port=3
  pointer : Inport  Port=4
  Add2 : Sum  Inputs=+|+|+|+|+
  Demux1 : Demux  Outputs=3
  If Action Subsystem : Subsystem  TreatAsAtomicUnit=on
  If Action Subsystem1 : Subsystem  TreatAsAtomicUnit=on
  If Action Subsystem2 : Subsystem  TreatAsAtomicUnit=on
  If Action Subsystem3 : Subsystem  TreatAsAtomicUnit=on
  If Action Subsystem4 : Subsystem  TreatAsAtomicUnit=on
  If Action Subsystem5 : Subsystem  TreatAsAtomicUnit=on
  If Action Subsystem6 : Subsystem  TreatAsAtomicUnit=on
  If Action Subsystem8 : Subsystem  TreatAsAtomicUnit=on
  If1 : If  NumInputs=2  IfExpression=u1>0 & u2>0
  If2 : If  NumInputs=2  IfExpression=u1<0 & u2>0
  If3 : If  NumInputs=2  IfExpression=u1>0 & u2<0
  If4 : If  NumInputs=2  IfExpression=u1<0 & u2<0
  Merge{,1..3} (4 alike) : Merge
  Reshape1 : Reshape  OutputDimensionality=Column vector (2-D)
  Terminator1 : Terminator
  creating distance between cm MB and centro geom lato : Subsystem
  Out1 : Outport
  wires:
  [A_vect] -> If Action Subsystem2/1(Areas_vect)
  [A_vect] -> If Action Subsystem1/1(Areas_vect)
  [A_vect] -> If Action Subsystem4/1(Areas_vect)
  Add2/1 -> Out1/1
  Merge3/1 -> Add2/5  "raggio vettore centro geom lato- centro geom lato illuminato"
  If4/1 -> If Action Subsystem2/Action
  If Action Subsystem2/1(r_cface_cluce_yneg_z_neg) -> Merge3/1
  If3/1 -> If Action Subsystem1/Action
  [A_vect] -> If Action Subsystem/1(Areas_vect)
  Merge1/1 -> Add2/3  "raggio vettore centro geom lato- centro geom lato illuminato"
  If Action Subsystem4/1(r_cface_cluce_zneg_y_pos) -> Merge1/1
  Merge/1 -> Add2/2  "raggio vettore centro geom lato- centro geom lato illuminato"
  If Action Subsystem/1(r_cface_cluce_yz_pos) -> Merge/1
  If1/2 -> If Action Subsystem8/Action
  S_B/1 -> Reshape1/1
  Reshape1/1 -> Demux1/1
  Demux1/2 -> If2/2, If3/2, If4/2, If1/2  "S_B_y"
  If2/1 -> If Action Subsystem4/Action
  If1/1 -> If Action Subsystem/Action
  Demux1/3 -> If4/1, If3/1, If2/1, If1/1  "S_B_z"
  creating distance between cm MB and centro geom lato/1(Out1) -> Add2/1
  Demux1/1 -> Terminator1/1  "S_B_x"
  MB/1 -> [MB]
  [MB] -> If Action Subsystem/2(MB)
  [MB] -> If Action Subsystem4/2(MB)
  [MB] -> If Action Subsystem1/2(MB)
  [MB] -> If Action Subsystem2/2(MB)
  If Action Subsystem8/1(Out1) -> Merge/2
  If2/2 -> If Action Subsystem3/Action
  If3/2 -> If Action Subsystem5/Action
  If4/2 -> If Action Subsystem6/Action
  If Action Subsystem3/1(Out1) -> Merge1/2
  If Action Subsystem1/1(r_cface_cluce_yneg_z_pos) -> Merge2/1
  If Action Subsystem5/1(Out1) -> Merge2/2
  Merge2/1 -> Add2/4  "raggio vettore centro geom lato- centro geom lato illuminato"
  If Action Subsystem6/1(Out1) -> Merge3/2
  [MB] -> creating distance between cm MB and centro geom lato/1(MB)
  A_vect/1 -> [A_vect]
  pointer/1 -> creating distance between cm MB and centro geom lato/2(pointer)

== system pointing_group24/Desturbances/External Torques/Solar radiation/Torque arm MB/creazione raggi vettore tra CM MB e centro facce illuminate della faccia che ha come normale l'asse j ==
  S_B : Inport
  MB : Inport  Port=2
  A_vect : Inport  Port=3
  pointer : Inport  Port=4
  Add2 : Sum  Inputs=+|+|+|+|+
  Demux1 : Demux  Outputs=3
  If Action Subsystem : Subsystem  TreatAsAtomicUnit=on
  If Action Subsystem1 : Subsystem  TreatAsAtomicUnit=on
  If Action Subsystem2 : Subsystem  TreatAsAtomicUnit=on
  If Action Subsystem3 : Subsystem  TreatAsAtomicUnit=on
  If Action Subsystem4 : Subsystem  TreatAsAtomicUnit=on
  If Action Subsystem5 : Subsystem  TreatAsAtomicUnit=on
  If Action Subsystem6 : Subsystem  TreatAsAtomicUnit=on
  If Action Subsystem7 : Subsystem  TreatAsAtomicUnit=on
  If1 : If  NumInputs=2  IfExpression=u1>0 & u2>0
  If2 : If  NumInputs=2  IfExpression=u1<0 & u2>0
  If3 : If  NumInputs=2  IfExpression=u1>0 & u2<0
  If4 : If  NumInputs=2  IfExpression=u1<0 & u2<0
  Merge{,1..3} (4 alike) : Merge
  Reshape1 : Reshape  OutputDimensionality=Column vector (2-D)
  Terminator1 : Terminator
  creating distance between cm MB and centro geom lato1 : Subsystem
  Out1 : Outport
  wires:
  Demux1/2 -> Terminator1/1
  creating distance between cm MB and centro geom lato1/1(Out1) -> Add2/1
  If1/1 -> If Action Subsystem/Action
  If2/1 -> If Action Subsystem1/Action
  Reshape1/1 -> Demux1/1
  S_B/1 -> Reshape1/1
  If Action Subsystem/1(r_cface_cluce_xz_pos) -> Merge/1
  Merge/1 -> Add2/2  "raggio vettore centro geom lato- centro geom lato illuminato"
  If Action Subsystem1/1(r_cface_cluce_x_pos_z_neg) -> Merge1/1
  Merge1/1 -> Add2/3  "raggio vettore centro geom lato- centro geom lato illuminato"
  [A_vect] -> If Action Subsystem/1(Areas_vect)
  Merge2/1 -> Add2/4  "raggio vettore centro geom lato- centro geom lato illuminato"
  If3/1 -> If Action Subsystem2/Action
  If Action Subsystem3/1(r_cface_cluce_x_neg_z_neg) -> Merge3/1
  If4/1 -> If Action Subsystem3/Action
  Merge3/1 -> Add2/5  "raggio vettore centro geom lato- centro geom lato illuminato"
  Add2/1 -> Out1/1
  [A_vect] -> If Action Subsystem1/1(Areas_vect)
  [A_vect] -> If Action Subsystem2/1(Areas_vect)
  [A_vect] -> If Action Subsystem3/1(Areas_vect)
  Demux1/3 -> If4/1, If3/1, If2/1, If1/1  "S_B_z"
  Demux1/1 -> If1/2, If4/2, If3/2, If2/2  "S_B_x"
  MB/1 -> [MB]
  [MB] -> If Action Subsystem/2(MB)
  [MB] -> If Action Subsystem1/2(MB)
  [MB] -> If Action Subsystem2/2(MB)
  [MB] -> If Action Subsystem3/2(MB)
  If1/2 -> If Action Subsystem5/Action
  If2/2 -> If Action Subsystem4/Action
  If3/2 -> If Action Subsystem6/Action
  If4/2 -> If Action Subsystem7/Action
  If Action Subsystem5/1(Out1) -> Merge/2
  If Action Subsystem4/1(Out1) -> Merge1/2
  If Action Subsystem2/1(r_cface_cluce_x_neg_z_pos) -> Merge2/1
  If Action Subsystem6/1(Out1) -> Merge2/2
  If Action Subsystem7/1(Out1) -> Merge3/2
  [MB] -> creating distance between cm MB and centro geom lato1/1(MB)
  A_vect/1 -> [A_vect]
  pointer/1 -> creating distance between cm MB and centro geom lato1/2(pointer)

== system pointing_group24/Desturbances/External Torques/Solar radiation/Torque arm MB/creazione raggi vettore tra CM MB e centro facce illuminate della faccia che ha come normale l'asse k ==
  S_B : Inport
  MB : Inport  Port=2
  A_vect : Inport  Port=3
  pointer : Inport  Port=4
  Add2 : Sum  Inputs=+|+|+|+|+
  Demux1 : Demux  Outputs=3
  If Action Subsystem : Subsystem  TreatAsAtomicUnit=on
  If Action Subsystem1 : Subsystem  TreatAsAtomicUnit=on
  If Action Subsystem2 : Subsystem  TreatAsAtomicUnit=on
  If Action Subsystem3 : Subsystem  TreatAsAtomicUnit=on
  If Action Subsystem4 : Subsystem  TreatAsAtomicUnit=on
  If Action Subsystem5 : Subsystem  TreatAsAtomicUnit=on
  If Action Subsystem6 : Subsystem  TreatAsAtomicUnit=on
  If Action Subsystem7 : Subsystem  TreatAsAtomicUnit=on
  If1 : If  NumInputs=2  IfExpression=u1>0 & u2>0
  If2 : If  NumInputs=2  IfExpression=u1<0 & u2>0
  If3 : If  NumInputs=2  IfExpression=u1>0 & u2<0
  If4 : If  NumInputs=2  IfExpression=u1<0 & u2<0
  Merge{,1..3} (4 alike) : Merge
  Reshape1 : Reshape  OutputDimensionality=Column vector (2-D)
  Terminator1 : Terminator
  creating distance between cm MB and centro geom lato1 : Subsystem
  Out1 : Outport
  wires:
  Demux1/3 -> Terminator1/1
  Demux1/1 -> If1/1, If4/1, If3/1, If2/1  "S_B_x"
  If1/1 -> If Action Subsystem/Action
  If2/1 -> If Action Subsystem4/Action
  Demux1/2 -> If4/2, If3/2, If2/2, If1/2  "S_B_y"
  Reshape1/1 -> Demux1/1
  S_B/1 -> Reshape1/1
  If1/2 -> If Action Subsystem5/Action
  Merge/1 -> Add2/2  "raggio vettore centro geom lato- centro geom lato illuminato"
  Merge1/1 -> Add2/3  "raggio vettore centro geom lato- centro geom lato illuminato"
  [A_vect] -> If Action Subsystem/1(Areas_vect)
  Merge2/1 -> Add2/4  "raggio vettore centro geom lato- centro geom lato illuminato"
  If3/2 -> If Action Subsystem6/Action
  If Action Subsystem1/1(r_cface_cluce_xpos_y_neg) -> Merge2/1
  If3/1 -> If Action Subsystem1/Action
  If4/2 -> If Action Subsystem7/Action
  If4/1 -> If Action Subsystem2/Action
  Merge3/1 -> Add2/5  "raggio vettore centro geom lato- centro geom lato illuminato"
  Add2/1 -> Out1/1
  [A_vect] -> If Action Subsystem4/1(Areas_vect)
  [A_vect] -> If Action Subsystem1/1(Areas_vect)
  [A_vect] -> If Action Subsystem2/1(Areas_vect)
  MB/1 -> [MB]
  [MB] -> If Action Subsystem/2(MB)
  [MB] -> If Action Subsystem4/2(MB1)
  [MB] -> If Action Subsystem1/2(MB)
  [MB] -> If Action Subsystem2/2(MB1)
  If2/2 -> If Action Subsystem3/Action
  If Action Subsystem/1(r_cface_cluce_xy_pos) -> Merge/1
  If Action Subsystem5/1(Out1) -> Merge/2
  If Action Subsystem4/1(r_cface_cluce_xneg_y_pos) -> Merge1/1
  If Action Subsystem3/1(Out1) -> Merge1/2
  If Action Subsystem6/1(Out1) -> Merge2/2
  If Action Subsystem2/1(r_cface_cluce_xneg_y_neg) -> Merge3/1
  If Action Subsystem7/1(Out1) -> Merge3/2
  [MB] -> creating distance between cm MB and centro geom lato1/1(MB)
  creating distance between cm MB and centro geom lato1/1(Out1) -> Add2/1
  A_vect/1 -> [A_vect]
  pointer/1 -> creating distance between cm MB and centro geom lato1/2(pointer)
